simulink model "rtwdemo_hyperlinks"  (Simulink 7.6)
settings: Solver=FixedStepDiscrete  StartTime=0.0  StopTime=48  FixedStep=1  RelTol=1e-3
libraries: rtwdemowidgets x2
Description:
  | Tracing Generated Code with Block / Code Highlighting
settings Model: Creator=The MathWorks Inc.  ParamWorkspaceSource=ReferencedWorkspace  CovMetricSettings=d  ExtModeTrigMode=oneshot  ExtModeArmWhenConnect=off  ExtModeAutoUpdateStatusClock=off
settings MATStruct: SampleTime=1  Offset=0  Priority=[20.0]
settings DataIOCC: LimitDataPoints=off  SaveFormat=StructureWithTime  SaveOutput=off  SaveTime=off  SignalLoggingName=sigsOut
settings OptimizationCC: InlineParams=on  InlineInvariantSignals=on  PassReuseOutputArgsAs=Individual arguments  StateBitsets=on  DataBitsets=on  UseTempVars=on  ZeroExternalMemoryAtStartup=off  ZeroInternalMemoryAtStartup=off  NoFixptDivByZeroProtection=on  EfficientFloat2IntCast=on  EfficientMapNaN2IntZero=off  OptimizeModelRefInitCode=on  LifeSpan=1
settings DebuggingCC: CheckExecutionContextPreStartOutputMsg=on  CheckExecutionContextRuntimeOutputMsg=on  SolverPrmCheckMsg=none  IntegerOverflowMsg=none  StrictBusMsg=ErrorOnBusTreatedAsVector
settings HardwareCC: ProdEndianess=LittleEndian  ProdHWDeviceType=Specified  TargetBitPerLong=64  TargetWordSize=64  TargetHWDeviceType=32-bit Generic
settings ModelReferenceCC: UpdateModelReferenceTargets=IfOutOfDate
settings SFSimCC: SimParseCustomCode=off
settings RTWCC: SystemTargetFile=ert.tlc  TLCOptions=-p0 -aWarnNonSaturatedBlocks=0  TemplateMakefile=ert_default_tmf  Description=Real-Time Workshop Embedded Coder (no auto configuration)  GenerateReport=on  RTWVerbose=off  ProcessScript=ert_make_rtw_hook  IncludeHyperlinkInReport=on  LaunchReport=on  GenerateTraceInfo=on  GenerateTraceReport=on  GenerateTraceReportSl=on  GenerateTraceReportSf=on  GenerateTraceReportEml=on
settings CodeAppCC: ForceParamTrailComments=on  IgnoreCustomStorageClasses=off  IgnoreTestpoints=on  SimulinkDataObjDesc=on  CustomSymbolStrGlobalVar=rt$N$M  CustomSymbolStrType=$N$M  CustomSymbolStrFcn=$N$M$F  CustomSymbolStrMacro=$N$M  InsertBlockDesc=on
settings ERTTargetCC: MultiwordLength=2048  GenerateSampleERTMain=on  IncludeMdlTerminateFcn=off  SupportNonFinite=off  SupportComplex=off  InlinedParameterPlacement=NonHierarchical  ERTCustomFileTemplate=example_file_process.tlc  ConvertIfToSwitch=off

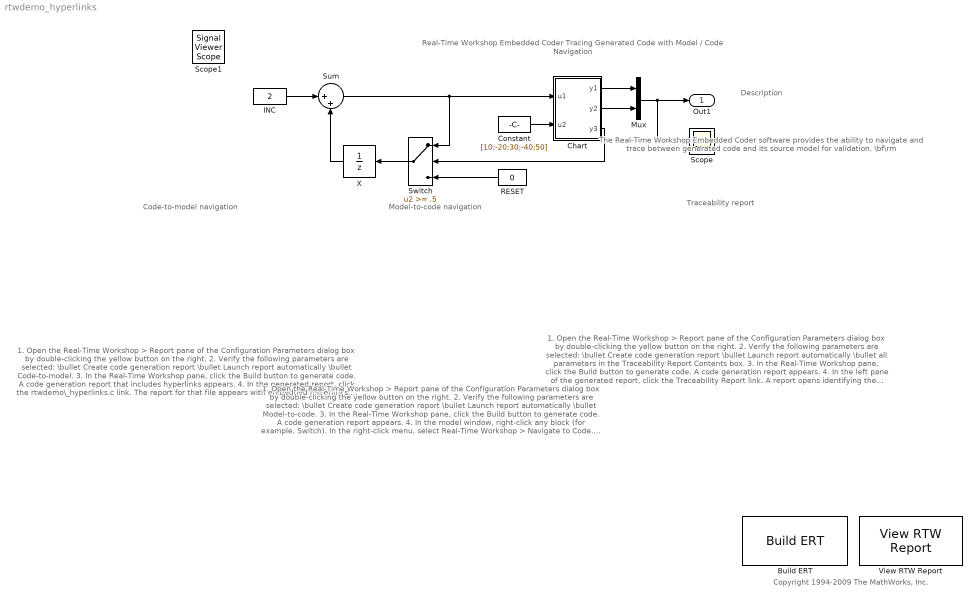
== system rtwdemo_hyperlinks ==
  note: Copyright 1994-2009 The MathWorks, Inc.
  note: Real-Time Workshop Embedded Coder
      | Tracing Generated Code with Model / Code Navigation
  note: Description
  note: The Real-Time Workshop Embedded Coder
      | software provides the ability to navigate and
      | trace between generated code and its source
      | model for validation.
      | \bf\rm
  note: Code-to-model navigation
  note: Model-to-code navigation
  note: 1. Open the Real-Time Workshop > Report pane
      |      of the Configuration Parameters dialog box by
      |      double-clicking the yellow button on the right.
      | 2. Verify the following parameters are selected:
      |     \bullet Create code generation report
      |     \bullet Launch report automatically
      |     \bullet Code-to-model.
      | 3. In the Real-Time Workshop pane, click the
      |     Build button to generate code. A code
      |     generation report that includes hyperlinks
      |     appears.
      | 4. In the generated report, click the
      |     rtwdemo\_hyperlinks.c link. The report for that
      |      file appears with embedded hyperlinks.
      | 5. Click various hyperlinks in the code. As you
      |     click each link, the corresponding portion
      |     of the model is highlighted. The highlighting
      |     helps you trace generated code segments
      |     back to the model. For example, if you click the
      |     hyperlink /* Sum: '<Root>/Sum' */, the Sum
      |     block in the model is highlighted.
      |
      | Double-clicking the blue button on the right
      | automates steps 1 through 3.
      | \bf\rm
  note: Traceability report
  note: 1. Open the Real-Time Workshop > Report pane of the
      |     Configuration Parameters dialog box by double-clicking
      |     the yellow button on the right.
      | 2. Verify the following parameters are selected:
      |     \bullet Create code generation report
      |     \bullet Launch report automatically
      |     \bullet all parameters in the Traceability Report
      |       Contents box.
      | 3. In the Real-Time Workshop pane, click the Build button
      |     to generate code. A code generation report appears.
      | 4. In the left pane of the generated report, click the
      |     Traceability Report link.  A report opens identifying the
      |     untraceable (not in the generated code) and traceable
      |     blocks in your model.
      | 5. In the traceability report, inspect the Eliminated /
      |     Virtual Blocks and Traceable Blocks lists.  For example,
      |     the Scope block is an untraceable block. It is listed
      |     under Eliminated / Virtual Blocks because the code
      |     generator does not create code for this block.
      |
      | Double-clicking the blue button on the right
      | automates steps 1 through 3.
      | \bf\rm
  note: 1. Open the Real-Time Workshop > Report pane of the
      |     Configuration Parameters dialog box by double-clicking
      |     the yellow button on the right.
      | 2. Verify the following parameters are selected:
      |    \bullet Create code generation report
      |    \bullet Launch report automatically
      |    \bullet Model-to-code.
      | 3. In the Real-Time Workshop pane, click the Build button
      |     to generate code.  A code generation report appears.
      | 4. In the model window, right-click any block (for example,
      |     Switch).  In the right-click menu,
      |     select Real-Time Workshop > Navigate to Code.
      |     Making this selection highlights the generated code
      |     for the block in the code generation report.
      | 5. Inspect the highlighted lines in the code generation
      |     report. The total number of highlighted lines is
      |     displayed next to each source file name in the left
      |     pane of the report.  Use the Previous and Next buttons
      |     to navigate through the highlighted lines.
      |
      | Double-clicking the blue button on the right automates
      | steps 1 through 3.
      |
      | \bfNote:\rm Model-to-code navigation also works for
      | Stateflow objects and Embedded MATLAB functions.
      |
      | \bfNote:\rm The report displays a diagnostic message
      | if there is no code to highlight for the selected
      | block (for example, if you select a virtual block).
      | \bf\rm
  Build ERT : rtwdemowidgets/Build ERT  SystemSampleTime=-1  attrib_overrides={}
  Chart : Stateflow chart  TreatAsAtomicUnit=on
  Constant : Constant  Value=[10;-20;30;-40;50]
  INC : Constant  Value=2  OutDataTypeStr=double
  Mux : Mux  Inputs=2
  RESET : Constant  Value=0  OutDataTypeStr=double
  Scope : Scope
  Sum : Sum  Inputs=|++  InputSameDT=on  OutDataTypeStr=Inherit: Same as first input
  Switch : Switch  Threshold=.5  SaturateOnIntegerOverflow=on  InputSameDT=on
  View RTW Report : rtwdemowidgets/View RTW Report  SystemSampleTime=-1
  X : UnitDelay  StateIdentifier=X
  Out1 : Outport
  Scope1 : SignalViewerScope  IOType=viewer  RefreshTime=0.035000
  wires:
  X/1 -> Sum/2
  Switch/1 -> X/1
  Sum/1 -> Chart/1(u1), Switch/1
  RESET/1 -> Switch/3
  INC/1 -> Sum/1
  Constant/1 -> Chart/2(u2)
  Chart/3(y3) -> Switch/2
  Chart/1(y1) -> Mux/1
  Chart/2(y2) -> Mux/2
  Mux/1 -> Out1/1, Scope/1

== stateflow chart Chart ==
  state S1
    en: loc= 2;
    ex: y3 = gfcn (u1, u2);
    state S1a [parallel]
      en: loc++;
      du: y1 = ttfcn(loc);
      settings: executionOrder=1
    state S1b [parallel]
      du: y2 = emfcn(u1, u2);
      settings: executionOrder=2
  state S2
    state S2a
      du: y1 = stgfcn(u1, u2);
      y2++;
    state S2b
      du: y1 = 2*(10+u2[0]);
    state out = stgfcn(in1, in2) [function]
      (default) -> (junction 13)
      (junction 13) -> (junction 14) [order 2] : {out = in2[1];}
      (junction 13) -> (junction 15) [order 1] : [in1>in2[1]]{out = in1;}
    S2a -> S2b : [after(3,tick)]
    (default) -> S2a
  state yg = gfcn(ug1, ug2) [function]
    (default) -> (junction 16) : {temp = ug1+ug2;}
    (junction 16) -> (junction 17) : {
        | yg = 10*(ug1+temp[0]+abs(ug2[1]));
        | }
  state yt = ttfcn(u1t) [function]
    (default) -> (junction 18)
    (junction 18) -> (junction 19) : { aVarTruthTableCondition_1 = ((u1t <= 0)); }
    (junction 19) -> (junction 20) : { aVarTruthTableCondition_2 = ((u1t > 0) && (u1t < 5)); }
    (junction 20) -> (junction 21) : { aVarTruthTableCondition_3 = ((u1t >= 5) && (u1t < 10)); }
    (junction 21) -> (junction 22) [order 1] : [aVarTruthTableCondition_1 && !aVarTruthTableCondition_2 && !aVarTruthTableCondition_3]
    (junction 22) -> (junction 23) : { yt = 10*(-1*u1t); }
    (junction 21) -> (junction 24) [order 2]
    (junction 24) -> (junction 25) [order 1] : [!aVarTruthTableCondition_1 && aVarTruthTableCondition_2 && !aVarTruthTableCondition_3]
    (junction 25) -> (junction 26) : { yt = 10*(u1t+5); }
    (junction 24) -> (junction 27) [order 2]
    (junction 27) -> (junction 28) [order 1] : [!aVarTruthTableCondition_1 && !aVarTruthTableCondition_2 && aVarTruthTableCondition_3]
    (junction 28) -> (junction 29) : { yt = 10*(u1t+10); }
    (junction 27) -> (junction 30) [order 2]
    (junction 30) -> (junction 31) : /* Default */
    (junction 31) -> (junction 32) : { yt = 100; }
  (default) -> S1
  S2 -> S1 : [after(2,tick)] {y3=0;
      |                         y1=0;}
  S1 -> S2 : [y1>50]
  data: in1 function_input double; in2 function_input double size=[5 1]; out function_output double; ug1 function_input double; ug2 function_input double size=[5 1]; yg function_output double; temp temporary double size=[5 1]; u1t function_input double; yt function_output double; aVarTruthTableCondition_1 temporary boolean =0; aVarTruthTableCondition_2 temporary boolean =0; aVarTruthTableCondition_3 temporary boolean =0; ye function_output double; u1e function_input double; u2e function_input double size=[5 1]; loc local double =-2; u1 input double; u2 input double size=[5 1]; y1 output double; y2 output double; y3 output double
  function ye = emfcn(u1e, u2e):
    | function ye = emfcn(u1e, u2e)
    |  
    | if (u1e > u2e(1))
    |     ye = power((abs(u2e(1)+ u2e(2))), 2) + u1e;
    | else
    |     ye = abs(u1e - u2e(2));
    | end
